simulink model "pwm_block2"  (R2015a)
settings: Solver=ode3  StartTime=0.0  StopTime=3  FixedStep=Ts  RelTol=1e-3
settings Model: Creator=rblan  LastModifiedBy=rblan

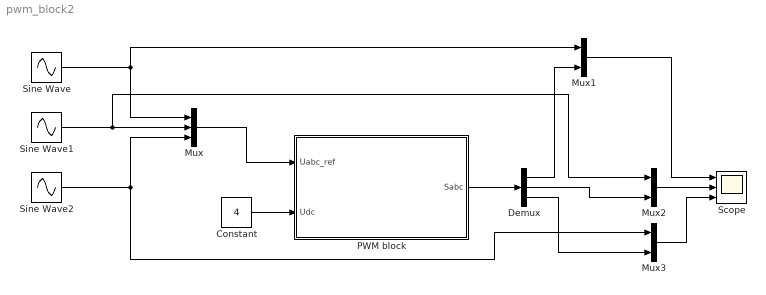
== system pwm_block2 ==
  Constant : Constant  Value=4
  Demux : Demux  Outputs=3
  Mux : Mux  Inputs=3
  Mux1 : Mux  Inputs=2
  Mux2 : Mux  Inputs=2
  Mux3 : Mux  Inputs=2
  PWM block : Subsystem
  Scope : Scope  NumInputPorts=3
      settings: YMin=-5~-5~-5  YMax=5~5~5
  Sine Wave : Sin  Frequency=50*2*pi  SampleTime=0
  Sine Wave1 : Sin  Frequency=50*2*pi  Phase=2*pi/3  SampleTime=0
  Sine Wave2 : Sin  Frequency=50*2*pi  Phase=4*pi/3  SampleTime=0
  wires:
  Constant/1 -> PWM block/2(Udc)
  Mux/1 -> PWM block/1(Uabc_ref)
  Sine Wave/1 -> Mux/1, Mux1/1
  Sine Wave1/1 -> Mux2/1, Mux/2
  Sine Wave2/1 -> Mux/3, Mux3/1
  Mux1/1 -> Scope/1
  PWM block/1(Sabc) -> Demux/1
  Demux/1 -> Mux1/2
  Mux2/1 -> Scope/2
  Demux/2 -> Mux2/2
  Mux3/1 -> Scope/3
  Demux/3 -> Mux3/2

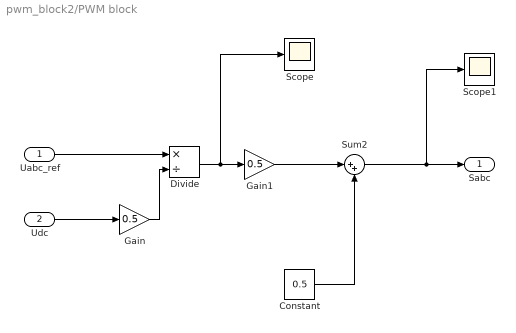
== system pwm_block2/PWM block ==
  Uabc_ref : Inport
  Udc : Inport  Port=2
  Constant : Constant  Value=0.5
  Divide : Product  Inputs=*/
  Gain : Gain  Gain=0.5
  Gain1 : Gain  Gain=0.5
  Scope : Scope
  Scope1 : Scope
      settings: SaveName=ScopeData2
  Sum2 : Sum  Inputs=|++
  Sabc : Outport
  wires:
  Udc/1 -> Gain/1
  Uabc_ref/1 -> Divide/1
  Gain/1 -> Divide/2
  Sum2/1 -> Scope1/1, Sabc/1
  Divide/1 -> Scope/1, Gain1/1
  Gain1/1 -> Sum2/1
  Constant/1 -> Sum2/2
